simulink model "TCAF_FTGSIM"  (R2022a)
settings: Solver=FixedStepDiscrete  StartTime=0.0  StopTime=2700  FixedStep=0.04  RelTol=1e-3
PreLoadFcn:
  | listing = dir;
  | if (contains([listing .name], 'TPF')) && (contains([listing .name], 'MAP'))
  |     addpath('./TCAF', './TRN', './FTG', './DYN', './FLCC', './GPS', './RALT', './INS', './MAP');
  | elseif (contains([listing .name], 'TCAF_WHOLESIM.slx'))
  |     addpath('./TCAF', './TRN', './FTG', '../DYN', '../FLCC', '../GPS', '../RALT', '../INS', '../MAP');
  | else
  | 
  | end
  | 
  | load('BUS_STRUCTURE_DYN.mat');
  | load('BUS_STRUCTURE_FLCC.mat');
  | load('BUS_STRUCTURE_RALT.mat');
  | load('BUS_STRUCTURE_INS.mat');
  | load('BUS_STRUCTURE_GPS.mat');
  | load('BusStructureTRN.mat');
  | load('BusStructureWTPG.mat');
  | load('BusStructureDTF.mat');
  | load('BusStructureGCAWS.mat');
InitFcn:
  | listing = dir;
  | if (contains([listing .name], 'TPF')) && (contains([listing .name], 'MAP'))
  |     addpath('./TCAF', './TRN', './FTG', './DYN', './FLCC', './GPS', './RALT', './INS', './MAP');
  | elseif (contains([listing .name], 'TCAF_WHOLESIM.slx'))
  |     addpath('./TCAF', './TRN', './FTG', '../DYN', '../FLCC', '../GPS', '../RALT', '../INS', '../MAP');
  | else
  | 
  | end
  | 
  | load('BUS_STRUCTURE_DYN.mat');
  | load('BUS_STRUCTURE_FLCC.mat');
  | load('BUS_STRUCTURE_RALT.mat');
  | load('BUS_STRUCTURE_INS.mat');
  | load('BUS_STRUCTURE_GPS.mat');
  | load('BusStructureTRN.mat');
  | load('BusStructureWTPG.mat');
  | load('BusStructureDTF.mat');
  | load('BusStructureGCAWS.mat');
settings Model: Creator=ASCL  LastModifiedBy=ASCL
settings SolverCC: PositivePriorityOrder=on
settings DataIOCC: ExternalInput=TCAF_WHOLESIMScenario.getElement('IN_TPF_WCPSIM_STICK'),TCAF_WHOLESIMScenario.getElement('IN_TPF_WCPSIM_FLIGHT_CMD'),TCAF_WHOLESIMScenario.getElement('IN_DTFIn'),TCAF_WHOLESIMScenario.getElement('IN_GCAWSIn')  SaveOutput=off  DSMLogging=off  ReturnWorkspaceOutputs=off
settings OptimizationCC: BlockReduction=off  DefaultParameterBehavior=Inlined  UseDivisionForNetSlopeComputation=on  GainParamInheritBuiltInType=on  UseFloatMulNetSlope=on  ExpressionFolding=off  PassReuseOutputArgsAs=Individual arguments  ZeroExternalMemoryAtStartup=off  ZeroInternalMemoryAtStartup=off  EfficientFloat2IntCast=on  LifeSpan=inf  OptimizeBlockOrder=speed  DifferentSizesBufferReuse=on  EfficientTunableParamExpr=on
settings DebuggingCC: SignalInfNanChecking=warning  ReadBeforeWriteMsg=EnableAllAsError  WriteAfterWriteMsg=EnableAllAsError  WriteAfterReadMsg=EnableAllAsError  IntegerOverflowMsg=error  ParameterTunabilityLossMsg=error  UniqueDataStoreMsg=error  AssertControl=DisableAll  NonBusSignalsTreatedAsBus=error  SFInvalidInputDataAccessInChartInitDiag=error  SFTransitionOutsideNaturalParentDiag=error  SFUnreachableExecutionPathDiag=error  SFUndirectedBroadcastEventsDiag=error  IntegerSaturationMsg=error
settings HardwareCC: ProdBitPerPointer=32  ProdBitPerSizeT=32  ProdBitPerPtrDiffT=32  ProdLargestAtomicInteger=Long  ProdLargestAtomicFloat=Double  ProdEndianess=BigEndian  ProdWordSize=32  ProdLongLongMode=on  ProdHWDeviceType=Freescale->MPC83xx
settings ModelReferenceCC: ModelReferenceNumInstancesAllowed=Single
settings SFSimCC: SimCustomHeaderCode="#include \"MAP.h\""  SimUserSources=MAP.c  SimUserLibraries=WS2_32.LIB  CompileTimeRecursionLimit=0  EnableRuntimeRecursion=off  MATLABDynamicMemAlloc=off
settings RTWCC: SystemTargetFile=ert.tlc  TemplateMakefile=ert_default_tmf  GenerateReport=on  RTWUseSimCustomCode=on  CustomHeaderCode="#include \"MAP.h\""  CustomSource=MAP.c  CustomLibrary=WS2_32.LIB  BuildConfiguration=Faster Runs  IncludeHyperlinkInReport=on  LaunchReport=on  GenerateTraceInfo=on  GenerateTraceReport=on  GenerateTraceReportSl=on  GenerateTraceReportSf=on  GenerateTraceReportEml=on
settings CodeAppCC: ForceParamTrailComments=on  IgnoreCustomStorageClasses=off  OperatorAnnotations=on  SimulinkDataObjDesc=on  SFDataObjDesc=on  MATLABFcnDesc=on  InsertBlockDesc=on  StateflowObjectComments=on  MATLABSourceComments=on  EnableCustomComments=on  InlinedPrmAccess=Macros  ReqsInCode=on
settings ERTTargetCC: TargetLangStandard=C99 (ISO)  UtilityFuncGeneration=Shared location  GenerateSampleERTMain=on  IncludeMdlTerminateFcn=off  CombineSignalStateStructs=on  SuppressErrorStatus=on  SupportAbsoluteTime=off  SupportNonFinite=off  SupportComplex=off  ParenthesesLevel=Standards  CastingMode=Standards  GenerateSharedConstants=off  InlinedParameterPlacement=NonHierarchical  ERTCustomFileTemplate=example_file_process.tlc  RateTransitionBlockCode=Function  PreserveIfCondition=on  ConvertIfToSwitch=off  EnableSignedLeftShifts=off  EnableSignedRightShifts=off

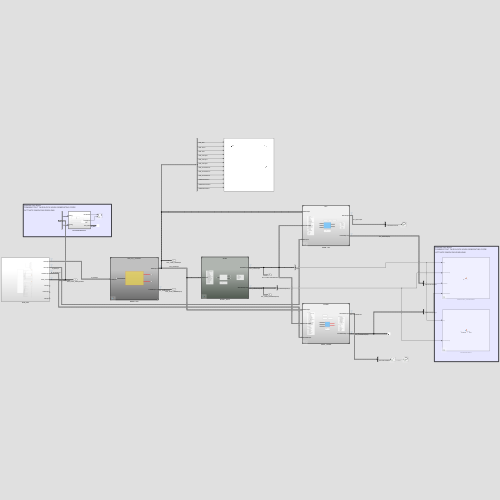
[thumbnail: Simulink's stored preview of the top-level diagram]
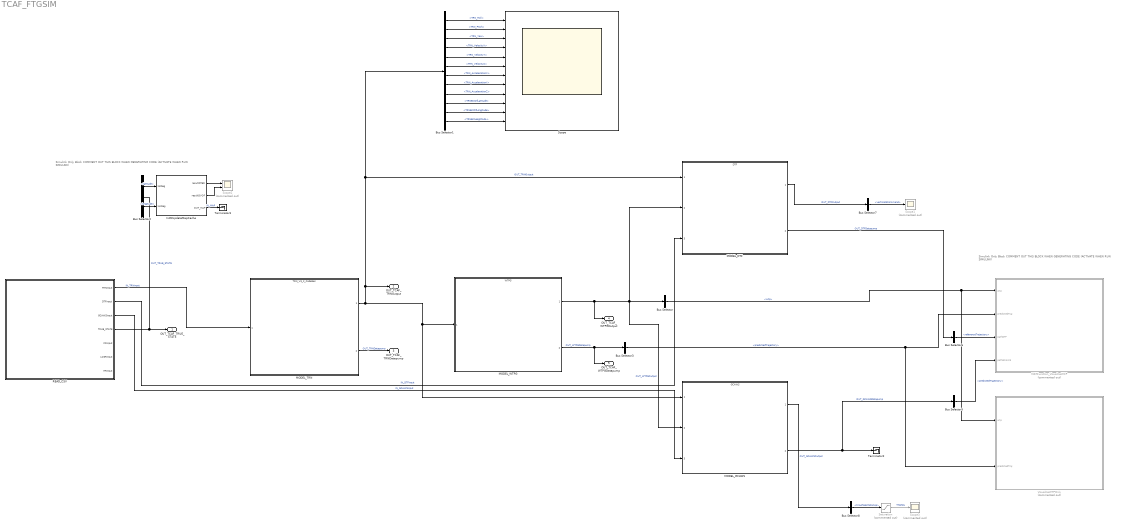
== system TCAF_FTGSIM ==
  note: Simulink Only Block
      | COMMENT OUT THIS BLOCK WHEN GENERATING CODE
      | (ACTIVATE WHEN RUN SIMULINK)
  note: Simulink Only Block
      | COMMENT OUT THIS BLOCK WHEN GENERATING CODE
      | (ACTIVATE WHEN RUN SIMULINK)
  Bus Selector : BusSelector  OutputSignals=wtp
  Bus Selector1 : BusSelector  OutputSignals=TRN_Roll,TRN_Pitch,TRN_Yaw,TRN_VelocityX,TRN_VelocityY,TRN_VelocityZ,TRN_AccelerationX,TRN_AccelerationY,TRN_AccelerationZ,TRNEstOfLatitude,TRNEstOfLongitude,TRNEstHeightAGL
  Bus Selector2 : BusSelector  OutputSignals=latitude,longitude
  Bus Selector3 : BusSelector  OutputSignals=predictedTrajectory
  Bus Selector5 : BusSelector  OutputSignals=predictedTrajectory
  Bus Selector6 : BusSelector  OutputSignals=referenceTrajectory
  Bus Selector7 : BusSelector  OutputSignals=verticalGCommand
  Bus Selector8 : BusSelector  OutputSignals=timeToGoToPullUp
  InitNUpdateMapCache : Subsystem  TreatAsAtomicUnit=on
  MATFunction_VisualizeWCP : MATLAB Function  Commented=on  TreatAsAtomicUnit=on
  MODEL_DTF : ModelReference  ModelNameDialog=DTF.slx  SimulationMode=Normal  ModelReferenceVersion=1.404
  MODEL_GCAWS : ModelReference  ModelNameDialog=GCAWS.slx  SimulationMode=Normal  ModelReferenceVersion=1.674
  MODEL_TRN : ModelReference  ModelNameDialog=TRN_V3_2_CodeGen.slx  SimulationMode=Normal  ModelReferenceVersion=2.325
  MODEL_WTPG : ModelReference  ModelNameDialog=WTPG.slx  SimulationMode=Normal  ModelReferenceVersion=1.309
  READ_CSV : Subsystem
  Saturation : Saturate  Commented=on  UpperLimit=5.0  LowerLimit=0.0
  Scope : Scope  NumInputPorts=12
  Scope1 : Scope  Commented=on
  Scope2 : Scope  Commented=on  NumInputPorts=2
  Scope3 : Scope  Commented=on
  Terminator2 : Terminator
  Terminator3 : Terminator
  VisualizeWTPOnly : MATLAB Function  Commented=on  TreatAsAtomicUnit=on
  OUT_TCAF_TRUE_STATE : Outport  OutDataTypeStr=Bus: BUS_DYN_STATE  BusOutputAsStruct=on
  OUT_TCAF_TRNOutput : Outport  Port=2  OutDataTypeStr=Bus: TRNOutput  BusOutputAsStruct=on
  OUT_TCAF_TRNDatapump : Outport  Port=3  OutDataTypeStr=Bus: TRNDatapump
  OUT_TCAF_WTPGOutput : Outport  Port=4  OutDataTypeStr=Bus: WTPGOutput
  OUT_TCAF_WTPGDatapump : Outport  Port=5  OutDataTypeStr=Bus: WTPGDatapump
  wires:
  Bus Selector7/1 -> Scope1/1  "<verticalGCommand>"
  Bus Selector6/1 -> MATFunction_VisualizeWCP/3(pathDTF)  "<referenceTrajectory>"
  Bus Selector1/4 -> Scope/4  "<TRN_VelocityX>"
  MODEL_DTF/2 -> Bus Selector6/1  "OUT_DTFDatapump"
  Bus Selector5/1 -> MATFunction_VisualizeWCP/4(pathGCAWS)  "<predictedTrajectory>"
  Bus Selector1/5 -> Scope/5  "<TRN_VelocityY>"
  InitNUpdateMapCache/3(OUT_MAP) -> Terminator3/1  "IN_MAP"
  Bus Selector1/7 -> Scope/7  "<TRN_AccelerationX>"
  Bus Selector1/8 -> Scope/8  "<TRN_AccelerationY>"
  MODEL_WTPG/1 -> OUT_TCAF_WTPGOutput/1, MODEL_GCAWS/2, MODEL_DTF/2, Bus Selector/1  "OUT_WTPGOutput"
  Bus Selector1/9 -> Scope/9  "<TRN_AccelerationZ>"
  Bus Selector1/12 -> Scope/12  "<TRNEstHeightAGL>"
  Bus Selector1/11 -> Scope/11  "<TRNEstOfLongitude>"
  MODEL_TRN/1 -> Bus Selector1/1, MODEL_DTF/1, OUT_TCAF_TRNOutput/1, MODEL_GCAWS/1, MODEL_WTPG/1  "OUT_TRNOutput"
  MODEL_WTPG/2 -> OUT_TCAF_WTPGDatapump/1, Bus Selector3/1  "OUT_WTPGDatapump"
  Bus Selector1/3 -> Scope/3  "<TRN_Yaw>"
  MODEL_GCAWS/2 -> Bus Selector5/1, Terminator2/1  "OUT_GCAWSDatapump"
  Bus Selector1/10 -> Scope/10  "<TRNEstOfLatitude>"
  MODEL_TRN/2 -> OUT_TCAF_TRNDatapump/1  "OUT_TRNDatapump"
  MODEL_GCAWS/1 -> Bus Selector8/1  "OUT_GCAWSOutput"
  Bus Selector1/6 -> Scope/6  "<TRN_VelocityZ>"
  Bus Selector3/1 -> VisualizeWTPOnly/2(predictedTraj), MATFunction_VisualizeWCP/2(predictedTraj)  "<predictedTrajectory>"
  InitNUpdateMapCache/1(resultDTED) -> Scope2/1
  READ_CSV/1(TRNInput) -> MODEL_TRN/1  "IN_TRNInput"
  Bus Selector/1 -> VisualizeWTPOnly/1(wtp), MATFunction_VisualizeWCP/1(wtp)  "<wtp>"
  Bus Selector1/1 -> Scope/1  "<TRN_Roll>"
  InitNUpdateMapCache/2(resultDVOF) -> Scope2/2
  MODEL_DTF/1 -> Bus Selector7/1  "OUT_DTFOutput"
  Bus Selector1/2 -> Scope/2  "<TRN_Pitch>"
  Bus Selector8/1 -> Saturation/1  "<timeToGoToPullUp>"
  Saturation/1 -> Scope3/1  "TTGTPU"
  READ_CSV/2(DTFInput) -> MODEL_DTF/3  "IN_DTFInput"
  READ_CSV/3(GCAWSInput) -> MODEL_GCAWS/3  "IN_GCAWSInput"
  READ_CSV/4(TRUE_STATE) -> OUT_TCAF_TRUE_STATE/1, Bus Selector2/1  "OUT_TRUE_STATE"
  Bus Selector2/1 -> InitNUpdateMapCache/1(latDeg)  "<latitude>"
  Bus Selector2/2 -> InitNUpdateMapCache/2(lonDeg)  "<longitude>"

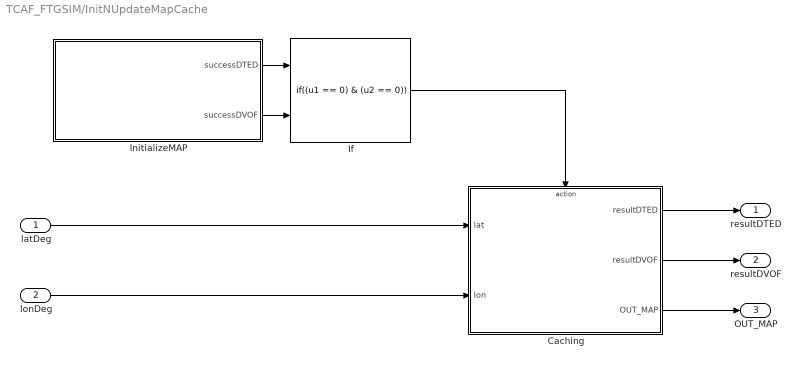
== system TCAF_FTGSIM/InitNUpdateMapCache ==
  latDeg : Inport  OutDataTypeStr=double
  lonDeg : Inport  Port=2  OutDataTypeStr=double
  Caching : Subsystem  TreatAsAtomicUnit=on
  If : If  NumInputs=2  IfExpression=(u1 == 0) & (u2 == 0)  ShowElse=off
  InitializeMAP : MATLAB Function  TreatAsAtomicUnit=on
  resultDTED : Outport  VectorParamsAs1DForOutWhenUnconnected=off
  resultDVOF : Outport  Port=2  VectorParamsAs1DForOutWhenUnconnected=off
  OUT_MAP : Outport  Port=3  OutDataTypeStr=Bus: TRN_MAP
  wires:
  lonDeg/1 -> Caching/2(lon)
  Caching/1(resultDTED) -> resultDTED/1
  InitializeMAP/1(successDTED) -> If/1
  latDeg/1 -> Caching/1(lat)
  Caching/2(resultDVOF) -> resultDVOF/1
  InitializeMAP/2(successDVOF) -> If/2
  If/1 -> Caching/Action
  Caching/3(OUT_MAP) -> OUT_MAP/1

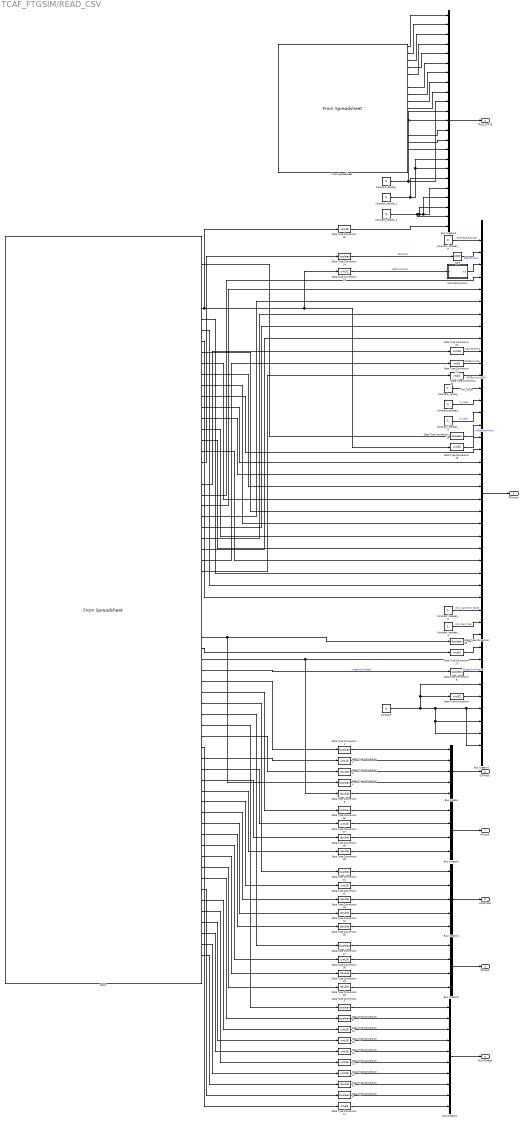
== system TCAF_FTGSIM/READ_CSV ==
  Bus Creator : BusCreator  Inputs=5  OutDataTypeStr=Bus: DTFInput  NonVirtualBus=on
      settings: InheritFromInputs=off
  Bus Creator1 : BusCreator  Inputs=10  OutDataTypeStr=Bus: GCAWSInput  NonVirtualBus=on
      settings: InheritFromInputs=off
  Bus Creator2 : BusCreator  Inputs=23  OutDataTypeStr=Bus: BUS_DYN_STATE  NonVirtualBus=on
      settings: InheritFromInputs=off
  Bus Creator3 : BusCreator  Inputs=4  OutDataTypeStr=Bus: CRInput  NonVirtualBus=on
      settings: InheritFromInputs=off
  Bus Creator4 : BusCreator  Inputs=5  OutDataTypeStr=Bus: LOSRInput  NonVirtualBus=on
      settings: InheritFromInputs=off
  Bus Creator5 : BusCreator  Inputs=4  OutDataTypeStr=Bus: HRInput  NonVirtualBus=on
      settings: InheritFromInputs=off
  Bus Creator7 : BusCreator  Inputs=42  OutDataTypeStr=Bus: TRNInput  NonVirtualBus=on
      settings: InheritFromInputs=off
  Constant : Constant  Value=0
  Constant_boolean_ : Constant  Value=0  OutDataTypeStr=boolean
  Constant_boolean_1 : Constant  OutDataTypeStr=boolean
  Constant_boolean_2 : Constant  OutDataTypeStr=boolean
  Constant_boolean_3 : Constant  OutDataTypeStr=boolean
  Constant_boolean_6 : Constant  Value=0  OutDataTypeStr=boolean
  Constant_double_ : Constant  Value=0  SampleTime=0.04
  Constant_double_1 : Constant  Value=0  SampleTime=0.04
  Constant_double_2 : Constant  Value=0  SampleTime=0.04
  Constant_uint16_ : Constant  OutDataTypeStr=uint16
  Data Type Conversion{,17..18,23} (4 alike) : DataTypeConversion  OutDataTypeStr=uint32  SaturateOnIntegerOverflow=off  RndMeth=Floor
  Data Type Conversion{1,4,6..9,19,24,26..27,31,36} (12 alike) : DataTypeConversion  OutDataTypeStr=boolean  RndMeth=Nearest  SaturateOnIntegerOverflow=off
  Data Type Conversion{3,5,10,28..29,33..35,38..39} (10 alike) : DataTypeConversion  OutDataTypeStr=double  RndMeth=Nearest  SaturateOnIntegerOverflow=off
  Data Type Conversion11 : DataTypeConversion  OutDataTypeStr=single  RndMeth=Nearest  SaturateOnIntegerOverflow=off
  Data Type Conversion{2,12..16,22,25,30,32,37} (11 alike) : DataTypeConversion  OutDataTypeStr=uint16  RndMeth=Nearest  SaturateOnIntegerOverflow=off
  Data Type Conversion20 : DataTypeConversion  OutDataTypeStr=int16  SaturateOnIntegerOverflow=off  RndMeth=Floor
  Data Type Conversion21 : DataTypeConversion  OutDataTypeStr=int16  SaturateOnIntegerOverflow=off  RndMeth=Floor
  From Spreadsheet : FromSpreadsheet  FileName=C:\Users\ASCL\Documents\DTNS\TC002_DTF\TRUE.csv  SheetName=TRUE  OutDataTypeStr=double  SampleTime=0.04  ExtrapolationBeforeFirstDataPoint=Hold first value  ExtrapolationAfterLastDataPoint=Hold last value
  INPUT : FromSpreadsheet  FileName=C:\Users\ASCL\Documents\DTNS\TC002_DTF\INPUT.csv  SheetName=INPUT  OutDataTypeStr=double  SampleTime=0.04  ExtrapolationBeforeFirstDataPoint=Hold first value  ExtrapolationAfterLastDataPoint=Hold last value
  MATLAB Function : MATLAB Function  TreatAsAtomicUnit=on
  NOT : Logic  Operator=NOT  IconShape=distinctive  AllPortsSameDT=off  OutDataTypeStr=boolean
  TRNInput : Outport  OutDataTypeStr=Bus: TRNInput
  DTFInput : Outport  Port=2  OutDataTypeStr=Bus: DTFInput
  GCAWSInput : Outport  Port=3  OutDataTypeStr=Bus: GCAWSInput
  TRUE_STATE : Outport  Port=4  OutDataTypeStr=Bus: BUS_DYN_STATE
  CRInput : Outport  Port=5  OutDataTypeStr=Bus: CRInput
  LOSRInput : Outport  Port=6  OutDataTypeStr=Bus: LOSRInput
  HRInput : Outport  Port=7  OutDataTypeStr=Bus: HRInput
  wires:
  Constant_double_2/1 -> Bus Creator2/20, Bus Creator2/19, Bus Creator2/21, Bus Creator2/22
  INPUT/10 -> Bus Creator7/22
  Data Type Conversion39/1 -> Bus Creator5/4
  INPUT/14 -> Bus Creator7/19
  From Spreadsheet/14 -> Bus Creator2/13
  From Spreadsheet/3 -> Bus Creator2/3
  From Spreadsheet/7 -> Bus Creator2/6
  From Spreadsheet/15 -> Bus Creator2/14
  From Spreadsheet/5 -> Bus Creator2/4
  From Spreadsheet/9 -> Bus Creator2/8
  Data Type Conversion38/1 -> Bus Creator5/3
  INPUT/45 -> Data Type Conversion11/1
  Data Type Conversion37/1 -> Bus Creator5/2
  Data Type Conversion12/1 -> Bus Creator1/3
  Data Type Conversion16/1 -> Bus Creator1/7
  Data Type Conversion36/1 -> Bus Creator5/1
  Data Type Conversion14/1 -> Bus Creator1/5
  INPUT/9 -> Bus Creator7/23
  Data Type Conversion13/1 -> Bus Creator1/4
  INPUT/13 -> Bus Creator7/18
  From Spreadsheet/4 -> Bus Creator2/5
  From Spreadsheet/8 -> Bus Creator2/7
  From Spreadsheet/16 -> Bus Creator2/15
  Constant_uint16_/1 -> Bus Creator7/13  "GPS_State"
  Data Type Conversion23/1 -> MATLAB Function/1(in)  "GPStimeValid"
  Bus Creator2/1 -> TRUE_STATE/1
  INPUT/29 -> Data Type Conversion20/1
  Constant_double_1/1 -> Bus Creator2/16, Bus Creator2/17, Bus Creator2/18
  INPUT/25 -> Bus Creator7/8
  Bus Creator/1 -> DTFInput/1
  INPUT/17 -> Bus Creator7/26
  From Spreadsheet/1 -> Bus Creator2/1
  INPUT/21 -> Data Type Conversion22/1
  Constant_boolean_/1 -> Bus Creator7/14  "C_code"
  INPUT/27 -> Bus Creator7/9
  INPUT/19 -> Data Type Conversion24/1
  INPUT/23 -> Bus Creator7/5
  INPUT/28 -> Data Type Conversion21/1
  INPUT/16 -> Bus Creator7/25
  INPUT/24 -> Bus Creator7/6
  Data Type Conversion6/1 -> Bus Creator7/36  "WieghtOnWheels"
  INPUT/22 -> Bus Creator7/4
  Data Type Conversion11/1 -> Bus Creator1/10
  INPUT/11 -> Bus Creator7/21
  INPUT/46 -> Data Type Conversion2/1
  INPUT/38 -> Data Type Conversion6/1  "WieghtOnWheels"
  INPUT/39 -> Data Type Conversion1/1
  Constant_boolean_2/1 -> Bus Creator7/31  "INS_Alignment_State"
  From Spreadsheet/2 -> Bus Creator2/2
  INPUT/62 -> Data Type Conversion14/1
  INPUT/58 -> Data Type Conversion9/1
  INPUT/60 -> Data Type Conversion15/1
  INPUT/63 -> Data Type Conversion16/1
  INPUT/59 -> Data Type Conversion12/1
  INPUT/61 -> Data Type Conversion13/1
  INPUT/57 -> Data Type Conversion8/1
  Data Type Conversion5/1 -> Bus Creator/5
  INPUT/64 -> Data Type Conversion10/1
  Data Type Conversion1/1 -> Bus Creator/1
  NOT/1 -> Bus Creator7/2  "GPSNotValid"
  Data Type Conversion/1 -> Bus Creator7/38
  INPUT/36 -> Data Type Conversion17/1
  INPUT/1 -> Data Type Conversion19/1
  Bus Creator7/1 -> TRNInput/1
  Data Type Conversion7/1 -> Bus Creator1/1
  Data Type Conversion10/1 -> Bus Creator1/8
  Constant_boolean_3/1 -> Bus Creator7/32  "INS_Mech_flag"
  INPUT/6 -> Bus Creator7/28
  Data Type Conversion9/1 -> Bus Creator1/9
  Data Type Conversion17/1 -> Bus Creator7/34
  Data Type Conversion19/1 -> Bus Creator7/16  "INSDataNotValid"
  INPUT/7 -> Bus Creator7/29
  INPUT/15 -> Bus Creator7/20
  Constant_boolean_6/1 -> Bus Creator7/1  "SoftResetRequest"
  Data Type Conversion21/1 -> Bus Creator7/11  "GPSEstHorlErr"
  Data Type Conversion22/1 -> Bus Creator7/10  "FigureOfMerit"
  Bus Creator1/1 -> GCAWSInput/1
  Data Type Conversion25/1 -> Bus Creator2/23
  Data Type Conversion26/1 -> Bus Creator7/33
  INPUT/8 -> Bus Creator7/30
  INPUT/12 -> Bus Creator7/24
  Data Type Conversion2/1 -> Bus Creator/2
  MATLAB Function/1(out) -> Bus Creator7/3
  Data Type Conversion20/1 -> Bus Creator7/12  "GPSEstVerticalErr"
  Data Type Conversion8/1 -> Bus Creator1/2
  Bus Creator3/1 -> CRInput/1
  Data Type Conversion27/1 -> Bus Creator3/1
  Data Type Conversion15/1 -> Bus Creator1/6
  INPUT/18 -> Bus Creator7/27
  Data Type Conversion28/1 -> Bus Creator3/4
  INPUT/26 -> Bus Creator7/7
  Data Type Conversion29/1 -> Bus Creator3/3
  Data Type Conversion18/1 -> Bus Creator7/17
  Data Type Conversion30/1 -> Bus Creator3/2
  Data Type Conversion4/1 -> Bus Creator/4
  Bus Creator4/1 -> LOSRInput/1
  Constant_boolean_1/1 -> Bus Creator7/15  "P_code"
  INPUT/51 -> Data Type Conversion33/1
  INPUT/55 -> Data Type Conversion29/1
  INPUT/50 -> Data Type Conversion32/1
  INPUT/54 -> Data Type Conversion30/1
  INPUT/41 -> Data Type Conversion31/1
  Data Type Conversion31/1 -> Bus Creator4/1
  Data Type Conversion32/1 -> Bus Creator4/2
  Data Type Conversion24/1 -> NOT/1  "GPSValid"
  Data Type Conversion3/1 -> Bus Creator/3
  Data Type Conversion33/1 -> Bus Creator4/3
  From Spreadsheet/10 -> Bus Creator2/9
  Data Type Conversion35/1 -> Bus Creator4/5
  Bus Creator5/1 -> HRInput/1
  INPUT/48 -> Data Type Conversion38/1
  INPUT/52 -> Data Type Conversion34/1
  INPUT/56 -> Data Type Conversion28/1
  INPUT/49 -> Data Type Conversion39/1
  INPUT/53 -> Data Type Conversion35/1
  INPUT/40 -> Data Type Conversion36/1
  INPUT/44 -> Data Type Conversion3/1
  INPUT/47 -> Data Type Conversion37/1
  INPUT/43 -> Data Type Conversion7/1
  Data Type Conversion34/1 -> Bus Creator4/4
  INPUT/42 -> Data Type Conversion27/1
  INPUT/37 -> Bus Creator7/35, Data Type Conversion5/1
  Constant_double_/1 -> Bus Creator2/12, Bus Creator2/11, Bus Creator2/10
  INPUT/35 -> Data Type Conversion26/1, Data Type Conversion4/1
  Constant/1 -> Bus Creator7/41, Bus Creator7/40, Bus Creator7/42, Bus Creator7/39, Data Type Conversion/1, Bus Creator7/37
  INPUT/5 -> Data Type Conversion18/1, Data Type Conversion23/1, Data Type Conversion25/1

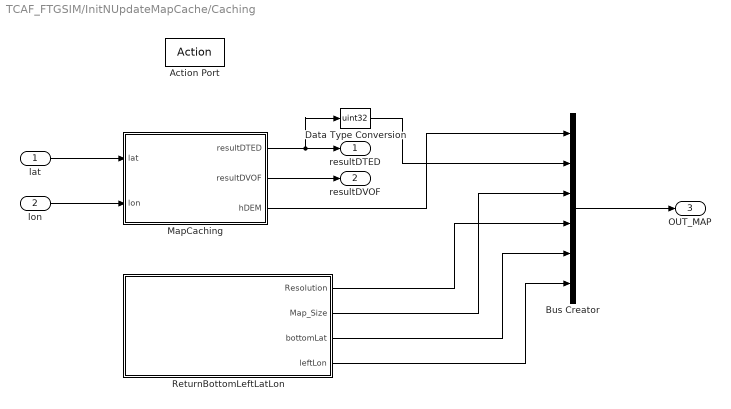
== system TCAF_FTGSIM/InitNUpdateMapCache/Caching ==
  lat : Inport
  lon : Inport  Port=2
  Action Port : ActionPort  ActionPortLabel=if((u1 == 0) & (u2 == 0))
  Bus Creator : BusCreator  Inputs=6  OutDataTypeStr=Bus: TRN_MAP  NonVirtualBus=on
  Data Type Conversion : DataTypeConversion  OutDataTypeStr=uint32  SaturateOnIntegerOverflow=off  RndMeth=Floor
  MapCaching : MATLAB Function  TreatAsAtomicUnit=on
  ReturnBottomLeftLatLon : MATLAB Function  TreatAsAtomicUnit=on
  resultDTED : Outport  VectorParamsAs1DForOutWhenUnconnected=off
  resultDVOF : Outport  Port=2  VectorParamsAs1DForOutWhenUnconnected=off
  OUT_MAP : Outport  Port=3  OutDataTypeStr=Bus: TRN_MAP
  wires:
  MapCaching/1(resultDTED) -> Data Type Conversion/1, resultDTED/1
  lat/1 -> MapCaching/1(lat)
  lon/1 -> MapCaching/2(lon)
  MapCaching/2(resultDVOF) -> resultDVOF/1
  Bus Creator/1 -> OUT_MAP/1
  ReturnBottomLeftLatLon/2(Map_Size) -> Bus Creator/3
  MapCaching/3(hDEM) -> Bus Creator/1
  ReturnBottomLeftLatLon/1(Resolution) -> Bus Creator/4
  ReturnBottomLeftLatLon/3(bottomLat) -> Bus Creator/5
  ReturnBottomLeftLatLon/4(leftLon) -> Bus Creator/6
  Data Type Conversion/1 -> Bus Creator/2

== matlab function TCAF_FTGSIM/InitNUpdateMapCache/Caching/ReturnBottomLeftLatLon ==
  data: Resolution output; Map_Size output; bottomLat output; leftLon output
function [Resolution, Map_Size, bottomLat, leftLon] = ReturnBottomLeftLatLon

Resolution = double(0.0);
Map_Size = double(0.0);

leftLon = 0.0;
leftLon = coder.ceval('ReturnLeftLon');

bottomLat = 0.0;
bottomLat = coder.ceval('ReturnBottomLat');

end

== matlab function TCAF_FTGSIM/MATFunction_VisualizeWCP ==
  data: wtp input; predictedTraj input; pathDTF input; pathGCAWS input
function Visualize(wtp, predictedTraj, pathDTF, pathGCAWS)
%VISUALIZE
% 
persistent fHandle subPlot1 subPlot2 tSpanWCP tSpanPT count map ARCSEC2DEG mapSurf predBound yAxisMax

acXY = zeros(2,27);
heading = 0;

% Initialize Figure Handle
if isempty(fHandle)
    fHandle = figure('WindowStyle', 'docked');
end

% Divide and Initailize the Figure
if isempty(subPlot1)
    set(0, 'CurrentFigure', fHandle);
    subPlot1 = subplot(1, 4, 1:2);
    axis equal;
    colormap(fliplr(hsv));
    view(0, 90);
    set(gca, 'Color', [0.3, 0.3, 0.3]);
    xlabel('Longitude [deg]');
    ylabel('Latitude [deg]');
    hold off;
end

% Divide and Initailize the Figure
if isempty(subPlot2)
    subPlot2 = subplot(1, 4, 3:4);
    hold on;
    grid minor;
    xlabel('Time [sec]');
    ylabel('Height [m]');
    axis([-0.5, 20, 0, 2000]);
    hold off;
end

% Initialize tSpanWCP
if isempty(tSpanWCP)
    tSpanWCP = 0:0.5:((length(wtp)-1)*0.5);
end

% Initialize tSpanPT
if isempty(tSpanPT)
    tSpanPT = 0:0.25:((size(predictedTraj, 1)-1)*0.25);
end

% Initialize count
if isempty(count)
    count = 0;    
end

% Initialize yAxisMax
if isempty(yAxisMax) 
    yAxisMax = 2000;
end
% Initialize ARCSEC2DEG
if isempty(ARCSEC2DEG)
    ARCSEC2DEG = (0.000277777777777777);
end

% Initialize map
if isempty(map)
    map = ones(150, 150, 3);

    % Current A/C Position
    latTrue = predictedTraj(1, 1, 1);
    lonTrue = predictedTraj(1, 1, 2);
    
    % Flooring to neighboring Map Grid
    latTrun = floor(latTrue/(3*ARCSEC2DEG)) * (3*ARCSEC2DEG);
    lonTrun = floor(lonTrue/(3*ARCSEC2DEG)) * (3*ARCSEC2DEG);
    
    mapSizeLat = size(map, 1);
    mapSizeLon = size(map, 2);
    % Update map data
    for ii = 1:size(map, 1)
    
        for jj = 1:size(map, 2)
            
            map(ii, jj, 1) = latTrun + (9*ARCSEC2DEG) * ((size(map, 1) - floor(mapSizeLat * 1.5)) + ii);
            map(ii, jj, 2) = lonTrun + (9*ARCSEC2DEG) * ((size(map, 2) - floor(mapSizeLon * 1.5)) + jj);
            
            map(ii, jj, 3) = ...
            coder.ceval('MAPGetTerrainHeight', map(ii, jj, 1), map(ii, jj, 2)); 

            if (ii == size(map, 1)) && (jj == size(map, 2))
                map(ii, jj, 3) = 2200;
            end
            
        end
    
    end
    
end

% Initialize mapSurf: mapSurf plot handle
if isempty(mapSurf)
    set(0, 'CurrentFigure', fHandle);
    subplot(subPlot1);
    hold on;
    mapSurf = surf(map(:,:,2), map(:,:,1), map(:,:,3), 'FaceAlpha', 0.75);
    drawnow;
    hold off;
end

% Initialize predBound: predBound plot handle
if isempty(predBound)
    set(0, 'CurrentFigure', fHandle);
    subplot(subPlot1);
    hold on;
    predBound = plot3([predictedTraj(:,2,2); flipud(predictedTraj(:,3,2))], ...
        [predictedTraj(:,2,1); flipud(predictedTraj(:,3,1))], ...
        [predictedTraj(:,2,3); flipud(predictedTraj(:,3,3))], '-m', 'LineWidth', 3);
    hold off;
end


%%

% Limit & Reset count
if (count >= 250)
    count = 0;
end

% 0.5Hz Event
if rem(count, 50) == 0
    set(0, 'CurrentFigure', fHandle);
    subplot(subPlot1);
    hold on;
    
    % Current A/C Position
    latTrue = predictedTraj(1, 1, 1);
    lonTrue = predictedTraj(1, 1, 2);
    
    % Flooring to neighboring Map Grid
    latTrun = floor(latTrue/(3*ARCSEC2DEG)) * (3*ARCSEC2DEG);
    lonTrun = floor(lonTrue/(3*ARCSEC2DEG)) * (3*ARCSEC2DEG);
    
    mapSizeLat = size(map, 1);
    mapSizeLon = size(map, 2);
    if abs(latTrun-(map(1, 1, 1)+map(end, 1, 1))/2) >= 100*(3*ARCSEC2DEG) || abs(lonTrun-(map(1, 1, 2)+map(1, end, 2))/2) >= 100*(3*ARCSEC2DEG)
        % Update map data
        for ii = 1:size(map, 1)
            for jj = 1:size(map, 2)
                map(ii, jj, 1) = latTrun + (9*ARCSEC2DEG) * ((size(map, 1) - floor(mapSizeLat * 1.5)) + ii);
                map(ii, jj, 2) = lonTrun + (9*ARCSEC2DEG) * ((size(map, 2) - floor(mapSizeLon * 1.5)) + jj);
                map(ii, jj, 3) = ...
                coder.ceval('MAPGetTerrainHeight', map(ii, jj, 1), map(ii, jj, 2)); 
            end
        end
        
        set(mapSurf, 'XData', map(:,:,2), 'YData', map(:,:,1), 'ZData', map(:,:,3));
        drawnow;
    end
    
    % Draw Map
    axis([lonTrun - (3*ARCSEC2DEG)*60, lonTrun + (3*ARCSEC2DEG)*60, latTrun - (3*ARCSEC2DEG)*60, latTrun + (3*ARCSEC2DEG)*60]);
    drawnow;
    hold off;
    
end

% 2.5Hz Event
if rem(count, 5) == 0
    set(0, 'CurrentFigure', fHandle);
    subplot(subPlot1);
    
    hold on;
    latTrue = predictedTraj(1, 1, 1);
    lonTrue = predictedTraj(1, 1, 2);
    heading = getHeadingFromVector([latTrue, lonTrue], [predictedTraj(81, 1, 1), predictedTraj(81, 1, 2)]);
    acXY = drawAircraft( [lonTrue;latTrue], 4.5*ARCSEC2DEG, heading);
    plot3(acXY(1,:), acXY(2,:), predictedTraj(1, 1, 3)*ones(size(acXY(1,:))), '-r')
    
    set(predBound, 'XData', [predictedTraj(:,2,2); flipud(predictedTraj(:,3,2))], ...
    'YData', [predictedTraj(:,2,1); flipud(predictedTraj(:,3,1))], ...
    'ZData', [predictedTraj(:,2,3); flipud(predictedTraj(:,3,3))]);
    
    hold off;
    
    set(0, 'CurrentFigure', fHandle);
    subplot(subPlot2);
    
    nominalTerrain = zeros(size(predictedTraj, 1), 1);
    for nn = 1:size(predictedTraj(:,1,3), 1)
        nominalTerrain(nn) = coder.ceval('MAPGetTerrainHeight', predictedTraj(nn, 1, 1), predictedTraj(nn, 1, 2)); 
    end
    
    hold on;
    cla
    plot(tSpanPT, nominalTerrain, '-g', 'LineWidth', 5, 'DisplayName', 'Nominal Terrain');
    plot(tSpanWCP, wtp, '-b', 'LineWidth', 5, 'DisplayName', 'WCP');
    plot(tSpanPT, predictedTraj(:, 1, 3), '--k', 'LineWidth', 2, 'DisplayName', 'Predicted Nominal Trajectory');
    plot(0, predictedTraj(1, 1, 3), 'ro', 'MarkerSize', 10, 'DisplayName', 'A/C');
    plot(0:0.5:20, pathDTF, '-y', 'DisplayName','DBTF Reference Trajectory', 'LineWidth', 2);
    
    for ii = 1:12
       plot(0:0.5:20, pathGCAWS(:,ii,3));
       
    end
    
    if (predictedTraj(1, 1, 3) > yAxisMax-300)
        axis([-0.5, 20, 0, predictedTraj(1, 1, 3) + 500]);
    elseif (predictedTraj(1, 1, 3) < 1800)
        axis([-0.5, 20, 0, 2000])
    end
    % axis([-1, 20, 300, 800]);
    drawnow;
    hold off; 
    
end

% Update count
count = count + 1;

end


function [acXY] = drawAircraft(centerXY, longLength, heading)
%DRAWAircraft
    % centerXY      (2x1)
    % longLength    (1) [deg]
    % heading       (1) [deg]
    
    acXY = zeros(2, 27);
    translate = ones(2, 27);
    translate(1,:) = translate(1,:) * centerXY(1); 
    translate(2,:) = translate(2,:) * centerXY(2); 
    
    refXY = [ 0, -2, -4, -6,-16,-16,-17,-17, -4, -4, -9,-10, -4,  0,  4, 10,  9,  4,  4, 17, 17, 16, 16,  6,  4,  2,  0;...
             25, 20,  8,  0, -7, -4, -4,-14,-14,-18,-23,-26,-25,-25,-25,-26,-23,-18,-14,-14, -4, -4, -7,  0,  8, 20, 25];
    
    acXY = refXY / 50 * longLength;
    
    rot = [cosd(-heading), -sind(-heading); sind(-heading), cosd(-heading)];
    
    acXY = rot * acXY + translate;
    
end

function [heading] = getHeadingFromVector(fromLatLon, toLatLon)
%GETHEADINGFROMVECTOR
    % fromLatLon (2x1) [deg]
    % toLatLon (2x1) [deg]
    
    dLon = toLatLon(2) - fromLatLon(2);
    
    y = sind(dLon) * cosd(toLatLon(1));
    x = cosd(fromLatLon(1)) * sind(toLatLon(1)) ...
        - sind(fromLatLon(1)) * cosd(toLatLon(1)) * cosd(dLon);
    
    heading = atan2d(y, x);
    heading = rem( heading + 360, 360);

end

== matlab function TCAF_FTGSIM/READ_CSV/MATLAB Function ==
  data: in input; out output
function out = fcn(in)
persistent count prevOut

if isempty(count)
    count = 0;
end
if isempty(prevOut)
    prevOut = uint32(0);
end

count = count + 1;

if mod(count, 25) == 0
    out = in;
    count = 0;
else
    out = prevOut;
end

prevOut = out;

== matlab function TCAF_FTGSIM/VisualizeWTPOnly ==
  data: wtp input; predictedTraj input
function VisualizeWTPOnly(wtp, predictedTraj)
%VisualizeWTPOnly
% 
persistent fHandle subPlot1 subPlot2 tSpanWCP tSpanPT count map ARCSEC2DEG mapSurf predBound yAxisMax

acXY = zeros(2,27);
heading = 0;

% Initialize Figure Handle
if isempty(fHandle)
    fHandle = figure('WindowStyle', 'docked');
end

% Divide and Initailize the Figure
if isempty(subPlot1)
    set(0, 'CurrentFigure', fHandle);
%     subPlot1 = subplot(5, 1, 1:4, 'position', [0.05 0.525 0.9 0.425]);
    subPlot1 = subplot(1, 4, 1:2);
    axis equal;
    colormap(fliplr(hsv));
    view(0, 90);
    set(gca, 'Color', [0.3, 0.3, 0.3]);
    xlabel('Longitude [deg]');
    ylabel('Latitude [deg]');
    hold off;
end

% Divide and Initailize the Figure
if isempty(subPlot2)
%     subPlot2 = subplot(5, 1, 5, 'position', [0.1 0.05 0.8 0.425]);
    subPlot2 = subplot(1, 4, 3:4);
    hold on;
    grid minor;
    xlabel('Time [sec]');
    ylabel('Height [m]');
    axis([-0.5, 20, 0, 2000]);
    hold off;
end

% Initialize tSpanWCP
if isempty(tSpanWCP)
    tSpanWCP = 0:0.5:((length(wtp)-1)*0.5);
end

% Initialize tSpanPT
if isempty(tSpanPT)
    tSpanPT = 0:0.25:((size(predictedTraj, 1)-1)*0.25);
end

% Initialize count
if isempty(count)
    count = 0;    
end

% Initialize yAxisMax
if isempty(yAxisMax) 
    yAxisMax = 2000;
end
% Initialize ARCSEC2DEG
if isempty(ARCSEC2DEG)
    ARCSEC2DEG = (0.000277777777777777);
end

% Initialize map
if isempty(map)
    map = ones(150, 150, 3);

    % Current A/C Position
    latTrue = predictedTraj(1, 1, 1);
    lonTrue = predictedTraj(1, 1, 2);
    
    % Flooring to neighboring Map Grid
    latTrun = floor(latTrue/(3*ARCSEC2DEG)) * (3*ARCSEC2DEG);
    lonTrun = floor(lonTrue/(3*ARCSEC2DEG)) * (3*ARCSEC2DEG);
    
    mapSizeLat = size(map, 1);
    mapSizeLon = size(map, 2);
    % Update map data
    for ii = 1:size(map, 1)
    
        for jj = 1:size(map, 2)
            
            map(ii, jj, 1) = latTrun + (9*ARCSEC2DEG) * ((size(map, 1) - floor(mapSizeLat * 1.5)) + ii);
            map(ii, jj, 2) = lonTrun + (9*ARCSEC2DEG) * ((size(map, 2) - floor(mapSizeLon * 1.5)) + jj);
            
            map(ii, jj, 3) = ...
            coder.ceval('MAPGetTerrainHeight', map(ii, jj, 1), map(ii, jj, 2)); 
            if (ii == size(map, 1)) && (jj == size(map,2))
                map(ii, jj, 3) = 2000;
            end
            
        end
    
    end
    
end

% Initialize mapSurf: mapSurf plot handle
if isempty(mapSurf)
    set(0, 'CurrentFigure', fHandle);
    subplot(subPlot1);
    hold on;
    mapSurf = surf(map(:,:,2), map(:,:,1), map(:,:,3), 'FaceAlpha', 0.85);
    drawnow;
    hold off;
end

% Initialize predBound: predBound plot handle
if isempty(predBound)
    set(0, 'CurrentFigure', fHandle);
    subplot(subPlot1);
    hold on;
    predBound = plot3([predictedTraj(:,2,2); flipud(predictedTraj(:,3,2))], ...
        [predictedTraj(:,2,1); flipud(predictedTraj(:,3,1))], ...
        [predictedTraj(:,2,3); flipud(predictedTraj(:,3,3))], '-m', 'LineWidth', 3);
    hold off;
end


%%

% Limit & Reset count
if (count >= 250)
    count = 0;
end

% 5Hz Event
if rem(count, 5) == 0
    set(0, 'CurrentFigure', fHandle);
    subplot(subPlot1);
    hold on;
    
    % Current A/C Position
    latTrue = predictedTraj(1, 1, 1);
    lonTrue = predictedTraj(1, 1, 2);
    
    % Flooring to neighboring Map Grid
    latTrun = floor(latTrue/(3*ARCSEC2DEG)) * (3*ARCSEC2DEG);
    lonTrun = floor(lonTrue/(3*ARCSEC2DEG)) * (3*ARCSEC2DEG);
    
    mapSizeLat = size(map, 1);
    mapSizeLon = size(map, 2);
    if abs(latTrun-(map(1, 1, 1)+map(end, 1, 1))/2) >= 100*(3*ARCSEC2DEG) || abs(lonTrun-(map(1, 1, 2)+map(1, end, 2))/2) >= 100*(3*ARCSEC2DEG)
        % Update map data
        for ii = 1:size(map, 1)
            for jj = 1:size(map, 2)
                map(ii, jj, 1) = latTrun + (9*ARCSEC2DEG) * ((size(map, 1) - floor(mapSizeLat * 1.5)) + ii);
                map(ii, jj, 2) = lonTrun + (9*ARCSEC2DEG) * ((size(map, 2) - floor(mapSizeLon * 1.5)) + jj);
                map(ii, jj, 3) = ...
                coder.ceval('MAPGetTerrainHeight', map(ii, jj, 1), map(ii, jj, 2)); 
            end
        end
        
        set(mapSurf, 'XData', map(:,:,2), 'YData', map(:,:,1), 'ZData', map(:,:,3));
        drawnow;
    end
    
    % Draw Map
    axis([lonTrun - (3*ARCSEC2DEG)*60, lonTrun + (3*ARCSEC2DEG)*60, latTrun - (3*ARCSEC2DEG)*60, latTrun + (3*ARCSEC2DEG)*60]);
    drawnow;
    hold off;
    
end

% 2.5Hz Event
if rem(count, 5) == 0
    set(0, 'CurrentFigure', fHandle);
    subplot(subPlot1);
    
    hold on;
    latTrue = predictedTraj(1, 1, 1);
    lonTrue = predictedTraj(1, 1, 2);
    heading = getHeadingFromVector([latTrue, lonTrue], [predictedTraj(81, 1, 1), predictedTraj(81, 1, 2)]);
    acXY = drawAircraft( [lonTrue;latTrue], 4.5*ARCSEC2DEG, heading);
    plot3(acXY(1,:), acXY(2,:), predictedTraj(1, 1, 3)*ones(size(acXY(1,:))), '-r')
    
    set(predBound, 'XData', [predictedTraj(:,2,2); flipud(predictedTraj(:,3,2))], ...
    'YData', [predictedTraj(:,2,1); flipud(predictedTraj(:,3,1))], ...
    'ZData', [predictedTraj(:,2,3); flipud(predictedTraj(:,3,3))]+200);
    
    hold off;
    
    set(0, 'CurrentFigure', fHandle);
    subplot(subPlot2);
    
    nominalTerrain = zeros(size(predictedTraj, 1), 1);
    for nn = 1:size(predictedTraj(:,1,3), 1)
        nominalTerrain(nn) = coder.ceval('MAPGetTerrainHeight', predictedTraj(nn, 1, 1), predictedTraj(nn, 1, 2)); 
    end
    
    hold on;
    cla
    plot(tSpanPT, nominalTerrain, '-g', 'LineWidth', 5, 'DisplayName', 'Nominal Terrain');
    plot(tSpanWCP, wtp, '-b', 'LineWidth', 5, 'DisplayName', 'WCP');

    if (predictedTraj(1, 1, 3) > yAxisMax-300)
        axis([-0.5, 20, 0, predictedTraj(1, 1, 3) + 500]);
    elseif (predictedTraj(1, 1, 3) < 1800)
        axis([-0.5, 20, 0, 2000])
    end
    % axis([-1, 20, 300, 800]);
    drawnow;
    hold off; 
    
end

% Update count
count = count + 1;

end


function [acXY] = drawAircraft(centerXY, longLength, heading)
%DRAWAircraft
    % centerXY      (2x1)
    % longLength    (1) [deg]
    % heading       (1) [deg]
    
    acXY = zeros(2, 27);
    translate = ones(2, 27);
    translate(1,:) = translate(1,:) * centerXY(1); 
    translate(2,:) = translate(2,:) * centerXY(2); 
    
    refXY = [ 0, -2, -4, -6,-16,-16,-17,-17, -4, -4, -9,-10, -4,  0,  4, 10,  9,  4,  4, 17, 17, 16, 16,  6,  4,  2,  0;...
             25, 20,  8,  0, -7, -4, -4,-14,-14,-18,-23,-26,-25,-25,-25,-26,-23,-18,-14,-14, -4, -4, -7,  0,  8, 20, 25];
    
    acXY = refXY / 50 * longLength;
    
    rot = [cosd(-heading), -sind(-heading); sind(-heading), cosd(-heading)];
    
    acXY = rot * acXY + translate;
    
end

function [heading] = getHeadingFromVector(fromLatLon, toLatLon)
%GETHEADINGFROMVECTOR
    % fromLatLon (2x1) [deg]
    % toLatLon (2x1) [deg]
    
    dLon = toLatLon(2) - fromLatLon(2);
    
    y = sind(dLon) * cosd(toLatLon(1));
    x = cosd(fromLatLon(1)) * sind(toLatLon(1)) ...
        - sind(fromLatLon(1)) * cosd(toLatLon(1)) * cosd(dLon);
    
    heading = atan2d(y, x);
    heading = rem( heading + 360, 360);

end

== matlab function TCAF_FTGSIM/InitNUpdateMapCache/Caching/MapCaching ==
  data: resultDTED output; resultDVOF output; lat input; lon input; hDEM output
function [resultDTED, resultDVOF, hDEM] = MapCaching(lat, lon)

persistent latPrev lonPrev

if isempty(latPrev)
    latPrev = 0.0;
end
if isempty(lonPrev)
    lonPrev = 0.0;
end

resultDTED = int32(1);
resultDVOF = int32(1);
hDEM = double(0.0);

if ( abs(lat - latPrev) > 0.01 ) || ( abs(lon - lonPrev) > 0.01)
    resultDVOF = coder.ceval('UpdateObstList', lat, lon);
    resultDTED = coder.ceval('UpdateMapCache', lat, lon);
    latPrev = lat;
    lonPrev = lon;
else

hDEM = coder.ceval('GetElevation', lat, lon);

end

== matlab function TCAF_FTGSIM/InitNUpdateMapCache/InitializeMAP ==
  data: successDTED output; successDVOF output
function [successDTED, successDVOF] = InitializeMAP()
persistent firstRun

if isempty(firstRun)
    firstRun = true;
end

flagDTED = int32(1);
flagDVOF = int32(1);

if firstRun
    
    pathDTED = 'C:\Users\ASCL\Documents\GitHub\DTNS\MAP\MAP_DB\';
    pathDVOF = 'C:\Users\ASCL\Documents\GitHub\DTNS\MAP\DVOF\';
    
    strLenDTED = int32(strlength(pathDTED));
    strLenDVOF = int32(strlength(pathDVOF));
    
    flagDTED = coder.ceval('InitialMap', pathDTED, strLenDTED );
    flagDVOF = coder.ceval('InitDVOF', pathDVOF, strLenDVOF );
    
    successDTED = flagDTED;
    successDVOF = flagDVOF;

    firstRun = false;
else
    successDTED = int32(0);
    successDVOF = int32(0);
end
